simulink model "coba"  (R2020a)
settings: Solver=VariableStepAuto  StartTime=0.0  StopTime=10.0  RelTol=1e-3
values from neighbouring files (symbols this model uses):
  C = 2    [rlc.m]
  k = 20    [func.m]
  kd = 9    [func.m]
  L = 1    [rlc.m]
  R = 1    [rlc.m]
settings Model: Creator=Iwan  LastModifiedBy=Iwan

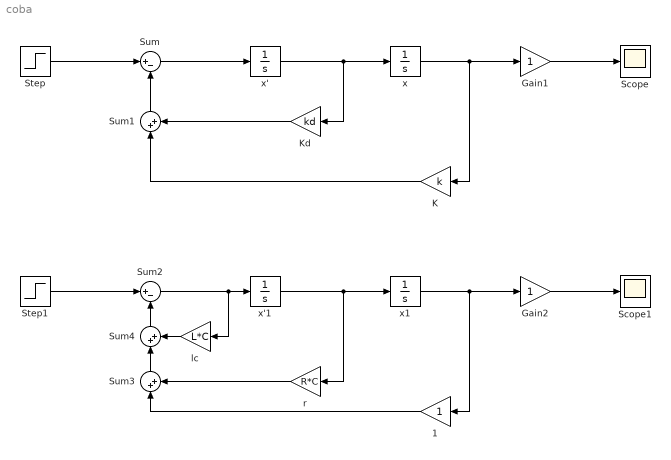
== system coba ==
  1 : Gain
  Gain1 : Gain
  Gain2 : Gain
  K : Gain  Gain=k
  Kd : Gain  Gain=kd
  Scope : Scope
  Scope1 : Scope
  Step : Step  Time=0  SampleTime=0
  Step1 : Step  Time=0  SampleTime=0
  Sum : Sum  Inputs=|+-
  Sum1 : Sum  Inputs=|++
  Sum2 : Sum  Inputs=|+-
  Sum3 : Sum  Inputs=|++
  Sum4 : Sum  Inputs=|++
  lc : Gain  Gain=L*C
  r : Gain  Gain=R*C
  x : Integrator
  x' : Integrator
  x'1 : Integrator
  x1 : Integrator
  wires:
  x/1 -> K/1, Gain1/1
  K/1 -> Sum1/1
  Kd/1 -> Sum1/2
  Sum1/1 -> Sum/2
  Gain1/1 -> Scope/1
  Sum/1 -> x'/1
  x'/1 -> Kd/1, x/1
  Step/1 -> Sum/1
  Step1/1 -> Sum2/1
  x'1/1 -> r/1, x1/1
  Sum2/1 -> lc/1, x'1/1
  Gain2/1 -> Scope1/1
  r/1 -> Sum3/2
  1/1 -> Sum3/1
  x1/1 -> 1/1, Gain2/1
  Sum3/1 -> Sum4/1
  Sum4/1 -> Sum2/2
  lc/1 -> Sum4/2
